simulink model "ADC"  (R2023a)
settings: Solver=VariableStepAuto  StartTime=0.0  StopTime=5  RelTol=1e-3
libraries: dspvision x1, dspsigops x1
settings Model: Creator=User  LastModifiedBy=User

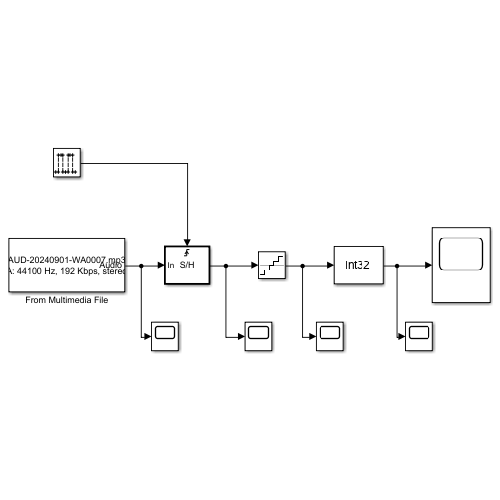
[thumbnail: Simulink's stored preview of the top-level diagram]
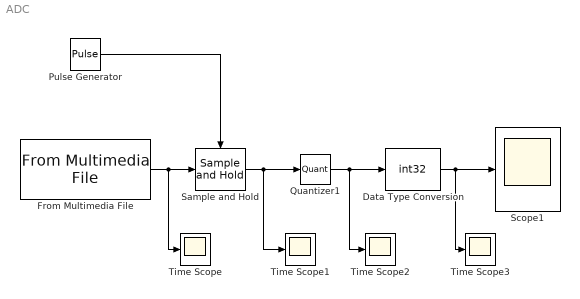
== system ADC ==
  Data Type Conversion : DataTypeConversion  OutDataTypeStr=int32  SaturateOnIntegerOverflow=off  RndMeth=Floor
  From Multimedia File : dspvision/From Multimedia File  inputFilename=C:\Users\User\Downloads\AUD-20240901-WA0007.mp3  readRange=[1 Inf]  loop=on  numPlays=inf  outputStreams=Audio only  videoDataType=single  audioDataType=double  inheritSampleTime=on  userDefinedSampleTime=1/30  noAudioOutput=off  isIntensityVideo=off  fourcc=RGB  colorVideoFormat=Separate color signals  outputEOF=off  dataOrg=Column-major  audioFrameSize=1024  computeAudioFrameSize=off  outSamplingMode=Sample based
      settings: LibrarySourceBlock=dspsrcs4/From Multimedia File
  Pulse Generator : DiscretePulseGenerator  Period=10  PulseWidth=5  SampleTime=0.01
  Quantizer1 : Quantizer  QuantizationInterval=0.25
  Sample and Hold : dspsigops/Sample and Hold  trig=Rising edge  initCond=0  latchinput=off
  Scope1 : Scope
  Time Scope{,1..3} (4 alike) : Scope
  wires:
  Pulse Generator/1 -> Sample and Hold/Trigger
  From Multimedia File/1 -> Time Scope/1, Sample and Hold/1
  Sample and Hold/1 -> Time Scope1/1, Quantizer1/1
  Data Type Conversion/1 -> Time Scope3/1, Scope1/1
  Quantizer1/1 -> Time Scope2/1, Data Type Conversion/1
